simulink model "magball_linear"  (R2018a)
settings: Solver=VariableStepAuto  StartTime=0.0  StopTime=2  RelTol=1e-3
settings Model: Creator=libingra  LastModifiedBy=libingra

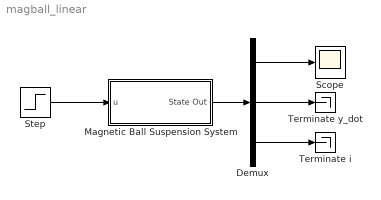
== system magball_linear ==
  Demux : Demux  Outputs=3
  Magnetic Ball Suspension System : Subsystem
  Scope : Scope
  Step : Step  Time=0  SampleTime=0
  Terminate i : Terminator
  Terminate y_dot : Terminator
  wires:
  Demux/2 -> Terminate y_dot/1
  Step/1 -> Magnetic Ball Suspension System/1(u)
  Magnetic Ball Suspension System/1(State Out) -> Demux/1
  Demux/1 -> Scope/1
  Demux/3 -> Terminate i/1

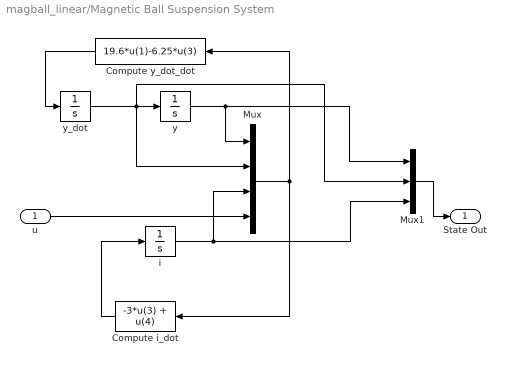
== system magball_linear/Magnetic Ball Suspension System ==
  u : Inport
  Compute i_dot : Fcn  Expr=-3*u(3) + u(4)
  Compute y_dot_dot : Fcn  Expr=19.6*u(1)-6.25*u(3)
  Mux : Mux
  Mux1 : Mux  Inputs=3
  i : Integrator
  y : Integrator
  y_dot : Integrator
  State Out : Outport
  wires:
  u/1 -> Mux/4
  Mux1/1 -> State Out/1
  y/1 -> Mux/1, Mux1/1
  y_dot/1 -> Mux1/2, Mux/2, y/1
  Compute y_dot_dot/1 -> y_dot/1
  Mux/1 -> Compute i_dot/1, Compute y_dot_dot/1
  Compute i_dot/1 -> i/1
  i/1 -> Mux1/3, Mux/3
